simulink library "VISMON_MASTER"  (Simulink 8.6)
settings: Solver=VariableStepAuto  StartTime=0.0  StopTime=10.0  RelTol=1e-3
libraries: VIS_LIB x21, VISMON_LIB x5, cdsMuxMatrix x5, cdsFilt x4, KAGRA_UTIL x3, cdsEpicsIn x1, cdsEpicsBinIn x1, cdsSqrt x1
settings Model: Creator=controls  LastModifiedBy=controls

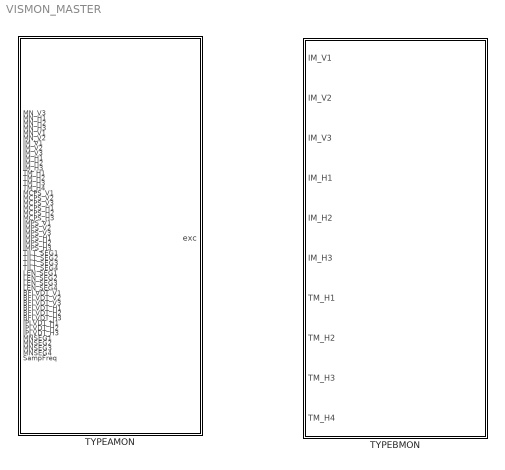
== system VISMON_MASTER ==
  TYPEAMON : Subsystem
  TYPEBMON : Subsystem

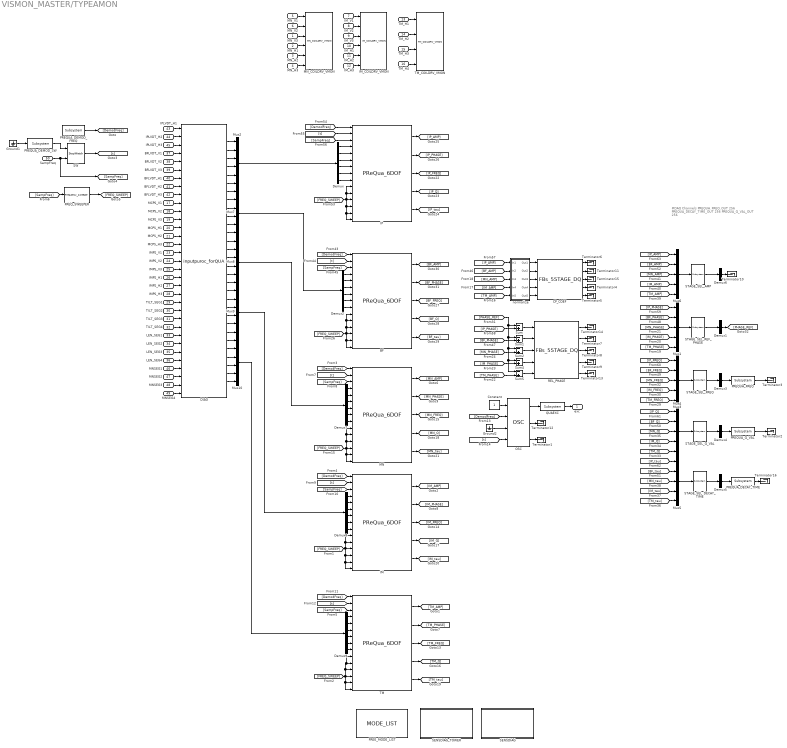
== system VISMON_MASTER/TYPEAMON ==
  note: #DAQ Channels
      |
      | PREQUA_FREQ_OUT 256
      | PREQUA_DECAY_TIME_OUT 256
      | PREQUA_Q_VAL_OUT 256
  MN_V3 : Inport
  MN_H1 : Inport  Port=2
  MN_H2 : Inport  Port=3
  MN_H3 : Inport  Port=4
  MN_V1 : Inport  Port=5
  MN_V2 : Inport  Port=6
  IM_V1 : Inport  Port=7
  IM_V2 : Inport  Port=8
  IM_V3 : Inport  Port=9
  IM_H1 : Inport  Port=10
  IM_H2 : Inport  Port=11
  IM_H3 : Inport  Port=12
  TM_H1 : Inport  Port=13
  TM_H2 : Inport  Port=14
  TM_H3 : Inport  Port=15
  TM_H4 : Inport  Port=16
  MCPS_V1 : Inport  Port=17
  MCPS_V2 : Inport  Port=18
  MCPS_V3 : Inport  Port=19
  MCPS_H1 : Inport  Port=20
  MCPS_H2 : Inport  Port=21
  MCPS_H3 : Inport  Port=22
  IMPS_V1 : Inport  Port=23
  IMPS_V2 : Inport  Port=24
  IMPS_V3 : Inport  Port=25
  IMPS_H1 : Inport  Port=26
  IMPS_H2 : Inport  Port=27
  IMPS_H3 : Inport  Port=28
  TILT_SEG1 : Inport  Port=29
  TILT_SEG2 : Inport  Port=30
  TILT_SEG3 : Inport  Port=31
  TILT_SEG4 : Inport  Port=32
  LEN_SEG1 : Inport  Port=33
  LEN_SEG2 : Inport  Port=34
  LEN_SEG3 : Inport  Port=35
  LEN_SEG4 : Inport  Port=36
  BFLVDT_V1 : Inport  Port=37
  BFLVDT_V2 : Inport  Port=38
  BFLVDT_V3 : Inport  Port=39
  BFLVDT_H1 : Inport  Port=40
  BFLVDT_H2 : Inport  Port=41
  BFLVDT_H3 : Inport  Port=42
  IPLVDT_H1 : Inport  Port=43
  IPLVDT_H2 : Inport  Port=44
  IPLVDT_H3 : Inport  Port=45
  MNSEG1 : Inport  Port=46
  MNSEG2 : Inport  Port=47
  MNSEG3 : Inport  Port=48
  MNSEG4 : Inport  Port=49
  SampFreq : Inport  Port=50
  BF : VIS_LIB/PReQua_6DOF
  CP_COEF : VIS_LIB/UTILs/FBs_5STAGE_DQ
  Constant : Constant
  DIAG : VIS_LIB/MODAL/inputpuroc_forQUA
  Demux{,2,7..9} (5 alike) : Demux  Outputs=6
  Demux{1,3..6} (5 alike) : Demux  Outputs=1
  FREE_MODE_LIST : VIS_LIB/MODE_LIST
  FREQ_SWEEPER : KAGRA_UTIL/Frequency_sweeper
  Ground1 : Ground
  Ground2 : Ground
  IM : VIS_LIB/PReQua_6DOF
  IM_COILDRV_VMON : VISMON_LIB/IM_COILDRV_VMON
  IP : VIS_LIB/PReQua_6DOF
  MN : VIS_LIB/PReQua_6DOF
  MN_COILDRV_VMON : VISMON_LIB/MN_COILDRV_VMON
  Mux{1,3..6} (5 alike) : Mux  Inputs=5
  Mux{2,7..10} (5 alike) : Mux  Inputs=6
  OSC : KAGRA_UTIL/pReQua_ver2/PLL/OSC
  PREQUA_DECAY_TIME : cdsFilt/Subsystem  Tag=cdsFilt  Description=|
      | Purpose:                                                                                                                                                                                                                                  
      | Standard CDS IIR filter module.                                                                                                                                                                                                           
      |                                                                                                                                                                                                                                           
      | Operation:                                                                                                                                                                                                                                
      | Consists of 10 second order section IIR filters, plus a ramped gain stage. In FE code, also provides pre-defined test points and excitation channel inputs. The filter coefficients are defined in the LIGO system using the 'foton' tool.
      |                                                                                                                                                                                                                                           
      | Usage:                                                                                                                                                                                                                                    
      | Name the part with the desired filter module name.
      settings: AttributesFormatString=%<Tag>
  PREQUA_DEMOD_FREQ : cdsEpicsIn/Subsystem  Tag=cdsEpicsIn  Description=|
      | Purpose:                                                                              
      | Create an EPICS input channel connection to the FE realtime controls.                 
      |                                                                                       
      | Operation:                                                                            
      | Outputs value from an EPICS ai record. Value is floating point with a precision of 3..
      |                                                                                       
      | Usage:                                                                                
      | Name the part with the desired EPICS channel name.
      settings: AttributesFormatString=%<Tag>
  PREQUA_DEMOD_SW : cdsEpicsBinIn/Subsystem  Tag=cdsEpicsBinIn  Description=|
      | Purpose:                                                                            
      | Create an EPICS binary (0 or 1) input channel to the FE realtime controls.          
      |                                                                                     
      | Operation:                                                                          
      | Outputs value from an EPICS ai record. Value is binary input (bi Epics record type).
      |                                                                                     
      | Usage:                                                                              
      | Name the part with the desired EPICS channel name.
      settings: AttributesFormatString=%<Tag>
  PREQUA_FREQ : cdsFilt/Subsystem  Tag=cdsFilt  Description=|
      | Purpose:                                                                                                                                                                                                                                  
      | Standard CDS IIR filter module.                                                                                                                                                                                                           
      |                                                                                                                                                                                                                                           
      | Operation:                                                                                                                                                                                                                                
      | Consists of 10 second order section IIR filters, plus a ramped gain stage. In FE code, also provides pre-defined test points and excitation channel inputs. The filter coefficients are defined in the LIGO system using the 'foton' tool.
      |                                                                                                                                                                                                                                           
      | Usage:                                                                                                                                                                                                                                    
      | Name the part with the desired filter module name.
      settings: AttributesFormatString=%<Tag>
  PREQUA_Q_VAL : cdsFilt/Subsystem  Tag=cdsFilt  Description=|
      | Purpose:                                                                                                                                                                                                                                  
      | Standard CDS IIR filter module.                                                                                                                                                                                                           
      |                                                                                                                                                                                                                                           
      | Operation:                                                                                                                                                                                                                                
      | Consists of 10 second order section IIR filters, plus a ramped gain stage. In FE code, also provides pre-defined test points and excitation channel inputs. The filter coefficients are defined in the LIGO system using the 'foton' tool.
      |                                                                                                                                                                                                                                           
      | Usage:                                                                                                                                                                                                                                    
      | Name the part with the desired filter module name.
      settings: AttributesFormatString=%<Tag>
  QUAEXC : cdsFilt/Subsystem  Tag=cdsFilt  Description=|
      | Purpose:                                                                                                                                                                                                                                  
      | Standard CDS IIR filter module.                                                                                                                                                                                                           
      |                                                                                                                                                                                                                                           
      | Operation:                                                                                                                                                                                                                                
      | Consists of 10 second order section IIR filters, plus a ramped gain stage. In FE code, also provides pre-defined test points and excitation channel inputs. The filter coefficients are defined in the LIGO system using the 'foton' tool.
      |                                                                                                                                                                                                                                           
      | Usage:                                                                                                                                                                                                                                    
      | Name the part with the desired filter module name.
      settings: AttributesFormatString=%<Tag>
  REL_PHASE : VIS_LIB/UTILs/FBs_5STAGE_DQ
  SENSDIAG : Subsystem
  SENSDIAG_TOWER : Subsystem
  STAGE_SEL_AMP : cdsMuxMatrix/Subsystem  Tag=cdsMuxMatrix  Description=Any size matrix. Inputs and outputs must be connected using Mux and Demux parts.
      settings: AttributesFormatString=%<Tag>
  STAGE_SEL_DECAY_TIME : cdsMuxMatrix/Subsystem  Tag=cdsMuxMatrix  Description=Any size matrix. Inputs and outputs must be connected using Mux and Demux parts.
      settings: AttributesFormatString=%<Tag>
  STAGE_SEL_FREQ : cdsMuxMatrix/Subsystem  Tag=cdsMuxMatrix  Description=Any size matrix. Inputs and outputs must be connected using Mux and Demux parts.
      settings: AttributesFormatString=%<Tag>
  STAGE_SEL_Q_VAL : cdsMuxMatrix/Subsystem  Tag=cdsMuxMatrix  Description=Any size matrix. Inputs and outputs must be connected using Mux and Demux parts.
      settings: AttributesFormatString=%<Tag>
  STAGE_SEL_REF_PHASE : cdsMuxMatrix/Subsystem  Tag=cdsMuxMatrix  Description=Any size matrix. Inputs and outputs must be connected using Mux and Demux parts.
      settings: AttributesFormatString=%<Tag>
  SW : KAGRA_UTIL/StopWatch
  Sum{,1..2,4..5} (5 alike) : Sum  Inputs=-+
  TM : VIS_LIB/PReQua_6DOF
  TM_COILDRV_VMON : VISMON_LIB/TM_COILDRV_VMON
  Terminator{1..16} (16 alike) : Terminator
  normalize : Subsystem
  exc : Outport
  wires:
  Mux10/1 -> Demux9/1
  Demux9/6 -> TM/9
  Demux9/5 -> TM/8
  Demux9/4 -> TM/7
  Demux9/3 -> TM/6
  Demux9/2 -> TM/5
  Demux9/1 -> TM/4
  DIAG/30 -> Mux10/6
  DIAG/29 -> Mux10/5
  DIAG/28 -> Mux10/4
  DIAG/27 -> Mux10/3
  DIAG/26 -> Mux10/2
  DIAG/25 -> Mux10/1
  Mux9/1 -> Demux8/1
  Demux8/6 -> IM/9
  Demux8/5 -> IM/8
  Demux8/4 -> IM/7
  Demux8/3 -> IM/6
  Demux8/2 -> IM/5
  Demux8/1 -> IM/4
  DIAG/24 -> Mux9/6
  DIAG/23 -> Mux9/5
  DIAG/22 -> Mux9/4
  DIAG/21 -> Mux9/3
  DIAG/20 -> Mux9/2
  DIAG/19 -> Mux9/1
  Mux8/1 -> Demux7/1
  DIAG/18 -> Mux8/6
  DIAG/17 -> Mux8/5
  DIAG/16 -> Mux8/4
  DIAG/15 -> Mux8/3
  DIAG/14 -> Mux8/2
  DIAG/13 -> Mux8/1
  Demux7/6 -> MN/9
  Demux7/5 -> MN/8
  Demux7/4 -> MN/7
  Demux7/3 -> MN/6
  Demux7/2 -> MN/5
  Demux7/1 -> MN/4
  Mux7/1 -> Demux2/1
  Demux2/6 -> BF/9
  Demux2/5 -> BF/8
  Demux2/4 -> BF/7
  Demux2/3 -> BF/6
  Demux2/2 -> BF/5
  Demux2/1 -> BF/4
  DIAG/12 -> Mux7/6
  DIAG/11 -> Mux7/5
  DIAG/10 -> Mux7/4
  DIAG/9 -> Mux7/3
  DIAG/8 -> Mux7/2
  DIAG/7 -> Mux7/1
  Demux/6 -> IP/9
  Demux/5 -> IP/8
  Demux/4 -> IP/7
  Demux/3 -> IP/6
  Demux/2 -> IP/5
  Demux/1 -> IP/4
  Mux2/1 -> Demux/1
  DIAG/6 -> Mux2/6
  DIAG/5 -> Mux2/5
  DIAG/4 -> Mux2/4
  DIAG/3 -> Mux2/3
  DIAG/2 -> Mux2/2
  DIAG/1 -> Mux2/1
  MNSEG4/1 -> DIAG/33
  MNSEG3/1 -> DIAG/32
  MNSEG1/1 -> DIAG/30
  MNSEG2/1 -> DIAG/31
  LEN_SEG4/1 -> DIAG/29
  LEN_SEG3/1 -> DIAG/28
  LEN_SEG2/1 -> DIAG/27
  LEN_SEG1/1 -> DIAG/26
  TILT_SEG4/1 -> DIAG/25
  TILT_SEG3/1 -> DIAG/24
  TILT_SEG2/1 -> DIAG/23
  TILT_SEG1/1 -> DIAG/22
  IMPS_H3/1 -> DIAG/21
  IMPS_H2/1 -> DIAG/20
  IMPS_H1/1 -> DIAG/19
  IMPS_V3/1 -> DIAG/18
  IMPS_V2/1 -> DIAG/17
  IMPS_V1/1 -> DIAG/16
  MCPS_H3/1 -> DIAG/15
  MCPS_H2/1 -> DIAG/14
  MCPS_H1/1 -> DIAG/13
  MCPS_V3/1 -> DIAG/12
  MCPS_V2/1 -> DIAG/11
  MCPS_V1/1 -> DIAG/10
  BFLVDT_H3/1 -> DIAG/9
  BFLVDT_H2/1 -> DIAG/8
  BFLVDT_H1/1 -> DIAG/7
  BFLVDT_V3/1 -> DIAG/6
  BFLVDT_V2/1 -> DIAG/5
  BFLVDT_V1/1 -> DIAG/4
  IPLVDT_H3/1 -> DIAG/3
  IPLVDT_H2/1 -> DIAG/2
  IPLVDT_H1/1 -> DIAG/1
  Demux6/1 -> Terminator10/1
  [IP_PHASE] -> Sum/2
  [BF_PHASE] -> Sum1/2
  [TM_PHASE] -> Sum5/2
  [IM_PHASE] -> Sum4/2
  [MN_PHASE] -> Sum2/2
  REL_PHASE/5 -> Terminator13/1
  REL_PHASE/4 -> Terminator9/1
  REL_PHASE/2 -> Terminator7/1
  REL_PHASE/1 -> Terminator14/1
  REL_PHASE/3 -> Terminator8/1
  CP_COEF/5 -> Terminator5/1
  CP_COEF/4 -> Terminator4/1
  CP_COEF/2 -> Terminator11/1
  CP_COEF/1 -> Terminator6/1
  CP_COEF/3 -> Terminator15/1
  [BF_AMP] -> normalize/2(In2)
  [IP_AMP] -> normalize/1(In1)
  [TM_AMP] -> normalize/5(In5)
  [IM_AMP] -> normalize/4(In4)
  [MN_AMP] -> normalize/3(In3)
  normalize/5(Out5) -> CP_COEF/5
  normalize/4(Out4) -> CP_COEF/4
  normalize/3(Out3) -> CP_COEF/3
  normalize/2(Out2) -> CP_COEF/2
  normalize/1(Out1) -> CP_COEF/1
  [IP_tau] -> Mux5/1
  [IP_Q] -> Mux4/1
  [IP_FREQ] -> Mux3/1
  [IP_PHASE] -> Mux1/1
  [IP_AMP] -> Mux6/1
  [IM_tau] -> Mux5/4
  [MN_tau] -> Mux5/3
  [BF_tau] -> Mux5/2
  [TM_Q] -> Mux4/5
  [IM_Q] -> Mux4/4
  [MN_Q] -> Mux4/3
  [BF_Q] -> Mux4/2
  [TM_FREQ] -> Mux3/5
  [IM_FREQ] -> Mux3/4
  [MN_FREQ] -> Mux3/3
  [BF_FREQ] -> Mux3/2
  [TM_PHASE] -> Mux1/5
  [IM_PHASE] -> Mux1/4
  [MN_PHASE] -> Mux1/3
  [BF_PHASE] -> Mux1/2
  [IM_AMP] -> Mux6/4
  [MN_AMP] -> Mux6/3
  [BF_AMP] -> Mux6/2
  [TM_AMP] -> Mux6/5
  BF/4 -> [BF_Q]
  BF/3 -> [BF_FREQ]
  BF/2 -> [BF_PHASE]
  BF/1 -> [BF_AMP]
  BF/5 -> [BF_tau]
  IP/4 -> [IP_Q]
  IP/3 -> [IP_FREQ]
  IP/2 -> [IP_PHASE]
  IP/1 -> [IP_AMP]
  IP/5 -> [IP_tau]
  Sum5/1 -> REL_PHASE/5
  [FREQ_SWEEP] -> IP/12, IP/13, IP/14, IP/15, IP/11, IP/10
  [SampFreq] -> IP/3
  [t] -> IP/2
  [DemodFreq] -> IP/1
  [TM_tau] -> Mux5/5
  Sum4/1 -> REL_PHASE/4
  [FREQ_SWEEP] -> BF/13, BF/14, BF/15, BF/12, BF/11, BF/10
  [SampFreq] -> BF/3
  [t] -> BF/2
  [DemodFreq] -> BF/1
  PREQUA_Q_VAL/1 -> Terminator2/1
  PREQUA_FREQ/1 -> Terminator3/1
  TM/5 -> [TM_tau]
  IM/5 -> [IM_tau]
  MN/5 -> [MN_tau]
  TM/4 -> [TM_Q]
  IM/4 -> [IM_Q]
  MN/4 -> [MN_Q]
  TM/3 -> [TM_FREQ]
  IM/3 -> [IM_FREQ]
  MN/3 -> [MN_FREQ]
  PREQUA_DECAY_TIME/1 -> Terminator16/1
  STAGE_SEL_AMP/1 -> Demux6/1
  Mux6/1 -> STAGE_SEL_AMP/1
  Demux5/1 -> PREQUA_DECAY_TIME/1
  STAGE_SEL_DECAY_TIME/1 -> Demux5/1
  Mux5/1 -> STAGE_SEL_DECAY_TIME/1
  Demux4/1 -> PREQUA_Q_VAL/1
  STAGE_SEL_Q_VAL/1 -> Demux4/1
  Mux4/1 -> STAGE_SEL_Q_VAL/1
  Demux3/1 -> PREQUA_FREQ/1
  STAGE_SEL_FREQ/1 -> Demux3/1
  Mux3/1 -> STAGE_SEL_FREQ/1
  Ground2/1 -> OSC/3
  Sum2/1 -> REL_PHASE/3
  Sum1/1 -> REL_PHASE/2
  Sum/1 -> REL_PHASE/1
  [PHASE_REF] -> Sum/1, Sum1/1, Sum2/1, Sum4/1, Sum5/1
  Demux1/1 -> [PHASE_REF]
  STAGE_SEL_REF_PHASE/1 -> Demux1/1
  Mux1/1 -> STAGE_SEL_REF_PHASE/1
  TM/2 -> [TM_PHASE]
  IM/2 -> [IM_PHASE]
  MN/2 -> [MN_PHASE]
  MN/1 -> [MN_AMP]
  IM/1 -> [IM_AMP]
  TM/1 -> [TM_AMP]
  [FREQ_SWEEP] -> TM/14, TM/15, TM/13, TM/12, TM/11, TM/10
  [FREQ_SWEEP] -> MN/13, MN/14, MN/15, MN/12, MN/11, MN/10
  [FREQ_SWEEP] -> IM/12, IM/13, IM/14, IM/15, IM/11, IM/10
  QUAEXC/1 -> exc/1
  OSC/1 -> QUAEXC/1
  OSC/3 -> Terminator1/1
  OSC/2 -> Terminator12/1
  Constant/1 -> OSC/1
  [t] -> OSC/4
  [DemodFreq] -> OSC/2
  Ground1/1 -> PREQUA_DEMOD_SW/1
  [SampFreq] -> FREQ_SWEEPER/1
  [SampFreq] -> TM/3
  [t] -> TM/2
  [DemodFreq] -> TM/1
  [SampFreq] -> IM/3
  [t] -> IM/2
  [DemodFreq] -> IM/1
  PREQUA_DEMOD_FREQ/1 -> [DemodFreq]
  FREQ_SWEEPER/1 -> [FREQ_SWEEP]
  [SampFreq] -> MN/3
  [t] -> MN/2
  [DemodFreq] -> MN/1
  SW/1 -> [t]
  SampFreq/1 -> SW/2, [SampFreq]
  PREQUA_DEMOD_SW/1 -> SW/1
  IM_H1/1 -> IM_COILDRV_VMON/4
  IM_H3/1 -> IM_COILDRV_VMON/6
  MN_H3/1 -> MN_COILDRV_VMON/6
  TM_H1/1 -> TM_COILDRV_VMON/1
  TM_H2/1 -> TM_COILDRV_VMON/2
  TM_H4/1 -> TM_COILDRV_VMON/4
  TM_H3/1 -> TM_COILDRV_VMON/3
  MN_V1/1 -> MN_COILDRV_VMON/1
  IM_H2/1 -> IM_COILDRV_VMON/5
  IM_V3/1 -> IM_COILDRV_VMON/3
  MN_V2/1 -> MN_COILDRV_VMON/2
  IM_V2/1 -> IM_COILDRV_VMON/2
  MN_V3/1 -> MN_COILDRV_VMON/3
  MN_H2/1 -> MN_COILDRV_VMON/5
  MN_H1/1 -> MN_COILDRV_VMON/4
  IM_V1/1 -> IM_COILDRV_VMON/1

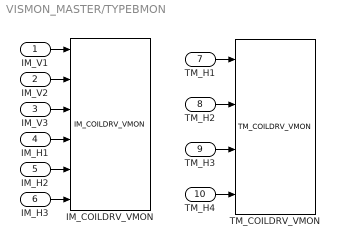
== system VISMON_MASTER/TYPEBMON ==
  IM_V1 : Inport
  IM_V2 : Inport  Port=2
  IM_V3 : Inport  Port=3
  IM_H1 : Inport  Port=4
  IM_H2 : Inport  Port=5
  IM_H3 : Inport  Port=6
  TM_H1 : Inport  Port=7
  TM_H2 : Inport  Port=8
  TM_H3 : Inport  Port=9
  TM_H4 : Inport  Port=10
  IM_COILDRV_VMON : VISMON_LIB/IM_COILDRV_VMON
  TM_COILDRV_VMON : VISMON_LIB/TM_COILDRV_VMON
  wires:
  IM_V1/1 -> IM_COILDRV_VMON/1
  IM_V2/1 -> IM_COILDRV_VMON/2
  IM_V3/1 -> IM_COILDRV_VMON/3
  IM_H2/1 -> IM_COILDRV_VMON/5
  TM_H3/1 -> TM_COILDRV_VMON/3
  TM_H4/1 -> TM_COILDRV_VMON/4
  TM_H2/1 -> TM_COILDRV_VMON/2
  TM_H1/1 -> TM_COILDRV_VMON/1
  IM_H3/1 -> IM_COILDRV_VMON/6
  IM_H1/1 -> IM_COILDRV_VMON/4

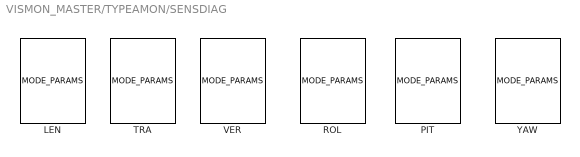
== system VISMON_MASTER/TYPEAMON/SENSDIAG ==
  LEN : VIS_LIB/MODE_PARAMS
  PIT : VIS_LIB/MODE_PARAMS
  ROL : VIS_LIB/MODE_PARAMS
  TRA : VIS_LIB/MODE_PARAMS
  VER : VIS_LIB/MODE_PARAMS
  YAW : VIS_LIB/MODE_PARAMS

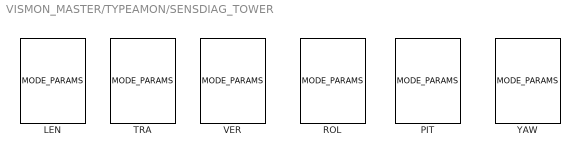
== system VISMON_MASTER/TYPEAMON/SENSDIAG_TOWER ==
  LEN : VIS_LIB/MODE_PARAMS
  PIT : VIS_LIB/MODE_PARAMS
  ROL : VIS_LIB/MODE_PARAMS
  TRA : VIS_LIB/MODE_PARAMS
  VER : VIS_LIB/MODE_PARAMS
  YAW : VIS_LIB/MODE_PARAMS

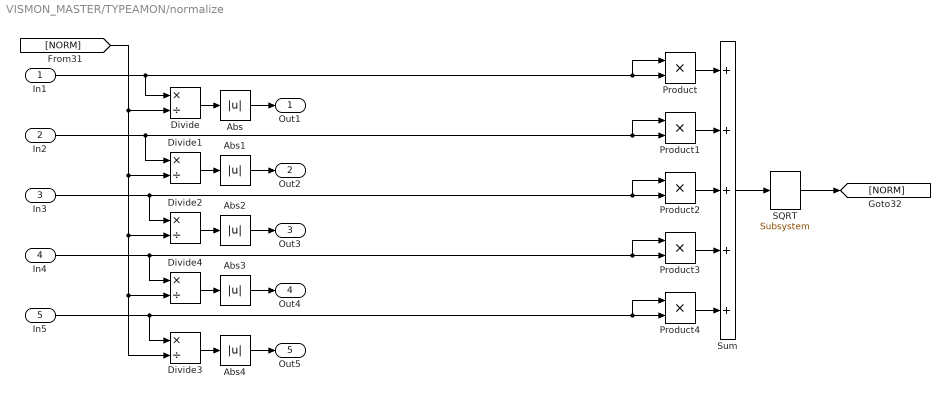
== system VISMON_MASTER/TYPEAMON/normalize ==
  In1 : Inport
  In2 : Inport  Port=2
  In3 : Inport  Port=3
  In4 : Inport  Port=4
  In5 : Inport  Port=5
  Abs{,1..4} (5 alike) : Abs
  Divide{,1..4} (5 alike) : Product  Inputs=*/
  Product{,1..4} (5 alike) : Product  RndMeth=Zero
  SQRT : cdsSqrt/Subsystem  Tag=cdsSqrt
      settings: AttributesFormatString=%<Tag>
  Sum : Sum  Inputs=+++++
  Out1 : Outport
  Out2 : Outport  Port=2
  Out3 : Outport  Port=3
  Out4 : Outport  Port=4
  Out5 : Outport  Port=5
  wires:
  Abs4/1 -> Out5/1
  Abs3/1 -> Out4/1
  Abs2/1 -> Out3/1
  Abs1/1 -> Out2/1
  Abs/1 -> Out1/1
  Product4/1 -> Sum/5
  Divide3/1 -> Abs4/1
  [NORM] -> Divide/2, Divide1/2, Divide2/2, Divide4/2, Divide3/2
  In5/1 -> Product4/2, Product4/1, Divide3/1
  Divide4/1 -> Abs3/1
  Product3/1 -> Sum/4
  In4/1 -> Product3/2, Product3/1, Divide4/1
  Divide2/1 -> Abs2/1
  Divide1/1 -> Abs1/1
  Divide/1 -> Abs/1
  In2/1 -> Product1/2, Product1/1, Divide1/1
  Product2/1 -> Sum/3
  Product/1 -> Sum/1
  Sum/1 -> SQRT/1
  In1/1 -> Product/2, Product/1, Divide/1
  Product1/1 -> Sum/2
  In3/1 -> Product2/2, Product2/1, Divide2/1
  SQRT/1 -> [NORM]
